simulink model "pwminverter"  (R2020a)
settings: Solver=VariableStepAuto  StartTime=0.0  StopTime=.05  RelTol=1e-3
libraries: powerlib x12, simulink x3, powerlib_meascontrol x1
settings Model: Creator=hp  LastModifiedBy=hp

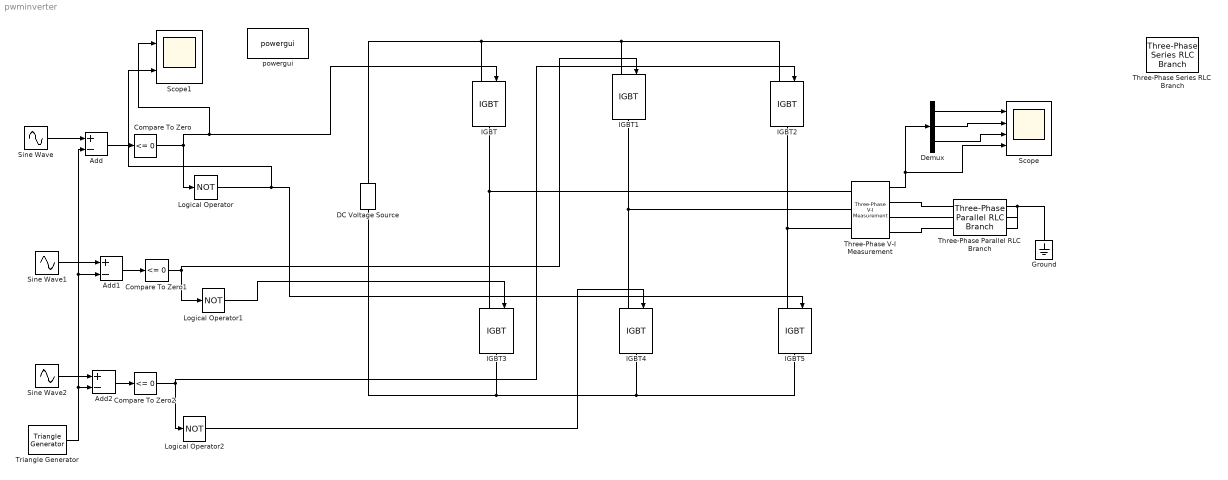
== system pwminverter ==
  Add : Sum  Inputs=+-
  Add1 : Sum  Inputs=+-
  Add2 : Sum  Inputs=+-
  Compare To Zero : simulink/Logic and Bit Operations/Compare To Zero  relop=<=  OutDataTypeStr=boolean
  Compare To Zero1 : simulink/Logic and Bit Operations/Compare To Zero  relop=<=  OutDataTypeStr=boolean
  Compare To Zero2 : simulink/Logic and Bit Operations/Compare To Zero  relop=<=  OutDataTypeStr=boolean
  DC Voltage Source : powerlib/Electrical Sources/DC Voltage Source  Amplitude=100  Measurements=None
  Demux : Demux  Outputs=3
  Ground : powerlib/Elements/Ground  LConnTagsString=a
  IGBT{,1..5} (6 alike) : powerlib/Power Electronics/IGBT  Ron=0.001  Lon=0  Vf=1  Tf=1e-6  Tt=2e-6  IC=0  Rs=1e5  Cs=inf  Measurements=off
  Logical Operator : Logic  Operator=NOT  Inputs=1  AllPortsSameDT=off  OutDataTypeStr=boolean
  Logical Operator1 : Logic  Operator=NOT  Inputs=1  AllPortsSameDT=off  OutDataTypeStr=boolean
  Logical Operator2 : Logic  Operator=NOT  Inputs=1  AllPortsSameDT=off  OutDataTypeStr=boolean
  Scope : Scope  NumInputPorts=4
  Scope1 : Scope  NumInputPorts=2
  Sine Wave : Sin  Frequency=2*pi*50  SampleTime=0
  Sine Wave1 : Sin  Frequency=2*pi*50  Phase=120*(pi/180)  SampleTime=0
  Sine Wave2 : Sin  Frequency=2*pi*50  Phase=240*(pi/180)  SampleTime=0
  Three-Phase Parallel RLC Branch : powerlib/Elements/Three-Phase Parallel RLC Branch  LConnTagsString=A|B|C  RConnTagsString=A|B|C  BranchType=R  Resistance=10  Inductance=1e-3  Capacitance=1e-6  Measurements=None
      settings: SourceProductBaseCode=PS
  Three-Phase Series RLC Branch : powerlib/Elements/Three-Phase Series RLC Branch  LConnTagsString=A|B|C  RConnTagsString=A|B|C  BranchType=R  Resistance=10  Inductance=1e-3  Capacitance=1e-6  Measurements=None
  Three-Phase V-I Measurement : powerlib/Measurements/Three-Phase V-I Measurement  VoltageMeasurement=phase-to-ground  SetLabelV=off  LabelV=Vabc  Vpu=off  VpuLL=off  CurrentMeasurement=no  SetLabelI=off  LabelI=Iabc  Ipu=off  Pbase=100e6  Vbase=500e3  OutputType=Complex  PhasorSimulation=off  PSBequivalent=0
  Triangle Generator : powerlib_meascontrol/Pulse & Signal Generators/Triangle Generator  Freq=100  Phase=90  Ts=0
  powergui : powerlib/powergui  Priority=1  SimulationMode=Discrete  SampleTime=50e-6  frequency=60  Iterations=50  frequencyindice=0  Pbase=100e6  ErrMax=1e-4  UnitsV=kV  UnitsW=MW  buscounter=0  FunctionMessages=off  echomessages=off  EnableUseOfTLC=off  CurrentSourceSwitches=off  DisableSnubberDevices=off  DisableRonSwitches=off  DisableVfSwitches=off  DisplayEquations=off  AutomaticDiscreteSolvers=off  SolverType=Tustin/Backward Euler (TBE)  Interpol=off  ExternalGateDelay=off  methode=off  Ts=100  x0status=blocks  SPID=on  SwTol=0  HookPort=off  NonlinearTolerance=1e-4  nMaxIteration=100  ContinueOnMaxIteration=off  RestoreLinks=warning  ResistiveCurrentMeasurement=off  Frange=[0:2:500]  Ylog=off  Xlog=on  ShowGrid=off  save=off  variable=ZData  structure=0  ZoomFFT=off  StartTime=0.0  cycles=1  DisplayStyle=1  fundamental=60  FreqAxis=off  MaxFrequency=1000  frequencyindicesteady=1  RmsSteady=1  display=off
  wires:
  Compare To Zero/1 -> Scope1/1, IGBT/1, Logical Operator/1
  Logical Operator/1 -> Scope1/2, IGBT5/1
  Compare To Zero1/1 -> IGBT1/1, Logical Operator1/1
  Logical Operator1/1 -> IGBT3/1
  Compare To Zero2/1 -> IGBT2/1, Logical Operator2/1
  Logical Operator2/1 -> IGBT4/1
  Triangle Generator/1 -> Add/2, Add1/2, Add2/2
  Sine Wave2/1 -> Add2/1
  Sine Wave1/1 -> Add1/1
  Sine Wave/1 -> Add/1
  Add2/1 -> Compare To Zero2/1
  Add1/1 -> Compare To Zero1/1
  Add/1 -> Compare To Zero/1
  Three-Phase V-I Measurement/1 -> Scope/4, Demux/1
  Demux/2 -> Scope/2
  Demux/1 -> Scope/1
  Demux/3 -> Scope/3
  connections:
  IGBT/RConn1 -- IGBT3/LConn1 -- Three-Phase V-I Measurement/LConn1
  IGBT1/RConn1 -- IGBT4/LConn1 -- Three-Phase V-I Measurement/LConn2
  IGBT2/RConn1 -- Three-Phase V-I Measurement/LConn3 -- IGBT5/LConn1
  DC Voltage Source/RConn1 -- IGBT/LConn1 -- IGBT1/LConn1 -- IGBT2/LConn1
  DC Voltage Source/LConn1 -- IGBT3/RConn1 -- IGBT4/RConn1 -- IGBT5/RConn1
  Three-Phase Parallel RLC Branch/LConn1 -- Three-Phase V-I Measurement/RConn1
  Three-Phase Parallel RLC Branch/LConn2 -- Three-Phase V-I Measurement/RConn2
  Three-Phase Parallel RLC Branch/LConn3 -- Three-Phase V-I Measurement/RConn3
  Three-Phase Parallel RLC Branch/RConn1 -- Three-Phase Parallel RLC Branch/RConn3 -- Three-Phase Parallel RLC Branch/RConn2 -- Ground/LConn1
